simulink model "Tariq"  (Simulink 10.0)
settings: Solver=ode45  StartTime=0.0  StopTime=10  RelTol=1e-3  EnableMultiTasking=on
undefined symbols (not defined in the file): B, f, J, Lm, Lr, Ls, P, Rr, Rs, Vm, We
libraries: simulink x2
settings Model: Creator=Administrator  LastModifiedBy=unknown
settings DataIOCC: LimitDataPoints=on  SignalLoggingSaveFormat=ModelDataLogs
settings OptimizationCC: ExpressionDepthLimit=2147483647  InitFltsAndDblsToZero=on
settings DebuggingCC: SaveWithParameterizedLinksMsg=none  SignalResolutionControl=TryResolveAllWithWarning  SolverPrmCheckMsg=warning  FcnCallInpInsideContextMsg=warning  StateNameClashWarn=warning
settings GRTTargetCC: TargetFcnLib=ansi_tfl_tmw.mat
settings ConfigComp: CovExternalEMLEnable=off

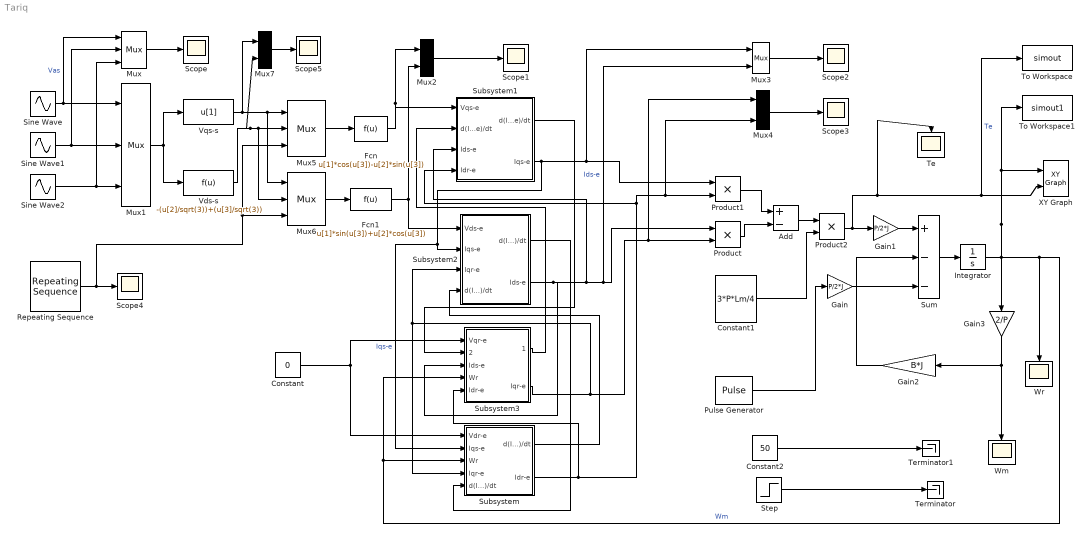
== system Tariq ==
  Add : Sum  Inputs=+-
  Constant : Constant  Value=0
  Constant1 : Constant  Value=3*P*Lm/4
  Constant2 : Constant  Value=50
  Fcn : Fcn  Expr=u[1]*cos(u[3])-u[2]*sin(u[3])
  Fcn1 : Fcn  Expr=u[1]*sin(u[3])+u[2]*cos(u[3])
  Gain : Gain  Gain=P/2*J
  Gain1 : Gain  Gain=P/2*J
  Gain2 : Gain  Gain=B*J
  Gain3 : Gain  Gain=2/P
  Integrator : Integrator
  Mux{,1,5..6} (4 alike) : Mux  Inputs=3
      settings: DisplayOption=signals
  Mux{2..4,7} (4 alike) : Mux  Inputs=2
      settings: DisplayOption=signals
  Product : Product  RndMeth=Zero
  Product1 : Product  RndMeth=Zero
  Product2 : Product  RndMeth=Zero
  Pulse Generator : DiscretePulseGenerator  Amplitude=40  Period=10  PulseWidth=5  PhaseDelay=4
  Repeating Sequence : simulink/Sources/Repeating Sequence  SystemSampleTime=-1  rep_seq_t=[0 1/f]  rep_seq_y=[0 2*pi]
  Scope{,1..5} (6 alike) : Scope
  Sine Wave : Sin  Amplitude=Vm  Frequency=2*pi*50  Phase=pi/2  SampleTime=0
  Sine Wave1 : Sin  Amplitude=Vm  Frequency=2*pi*50  Phase=(pi/2)-(2*pi/3)  SampleTime=0
  Sine Wave2 : Sin  Amplitude=Vm  Frequency=2*pi*50  Phase=(pi/2)+(2*pi/3)  SampleTime=0
  Step : Step  Time=0.5  After=40  SampleTime=0
  Subsystem : Subsystem
  Subsystem1 : Subsystem
  Subsystem2 : Subsystem
  Subsystem3 : Subsystem
  Sum : Sum  Inputs=+--
  Te : Scope
  Terminator : Terminator
  Terminator1 : Terminator
  To Workspace : ToWorkspace  VariableName=simout  SaveFormat=Structure  SampleTime=-1
  To Workspace1 : ToWorkspace  VariableName=simout1  SaveFormat=Structure  SampleTime=-1
  Vds-s : Fcn  Expr=-(u[2]/sqrt(3))+(u[3]/sqrt(3))
  Vqs-s : Fcn  Expr=u[1]
  Wm : Scope
  Wr : Scope
  XY Graph : simulink/Sinks/XY Graph  SystemSampleTime=-1  xmin=0  xmax=350  ymin=-400  ymax=400  st=-1
  wires:
  Mux/1 -> Scope/1
  Mux2/1 -> Scope1/1
  Mux3/1 -> Scope2/1
  Mux4/1 -> Scope3/1
  Product1/1 -> Add/1
  Product/1 -> Add/2
  Add/1 -> Product2/1
  Constant1/1 -> Product2/2
  Product2/1 -> Gain1/1, XY Graph/2, To Workspace/1, Te/1  "Te"
  Gain1/1 -> Sum/1
  Gain/1 -> Sum/3
  Pulse Generator/1 -> Gain/1
  Sum/1 -> Integrator/1
  Integrator/1 -> XY Graph/1, To Workspace1/1, Gain3/1, Subsystem3/4(Wr), Subsystem/3(Wr), Wr/1  "Wm"
  Gain2/1 -> Sum/2
  Gain3/1 -> Wm/1, Gain2/1
  Constant2/1 -> Terminator1/1
  Step/1 -> Terminator/1
  Repeating Sequence/1 -> Scope4/1, Mux5/3, Mux6/3
  Sine Wave/1 -> Mux1/1, Mux/1  "Vas"
  Sine Wave1/1 -> Mux1/2, Mux/2
  Sine Wave2/1 -> Mux1/3, Mux/3
  Mux1/1 -> Vqs-s/1, Vds-s/1
  Vqs-s/1 -> Mux5/1, Mux6/1, Mux7/1
  Vds-s/1 -> Mux5/2, Mux6/2, Mux7/2
  Mux5/1 -> Fcn/1
  Mux6/1 -> Fcn1/1
  Fcn/1 -> Mux2/1, Subsystem1/1(Vqs-e)
  Fcn1/1 -> Mux2/2, Subsystem2/1(Vds-e)
  Mux7/1 -> Scope5/1
  Subsystem1/2(Iqs-e) -> Subsystem2/2(Iqs-e), Subsystem/2(Iqs-e), Product1/1, Mux3/1  "Iqs-e"
  Subsystem/2(Idr-e) -> Subsystem1/4(Idr-e), Product1/2, Mux4/2, Subsystem3/5(Idr-e)
  Subsystem2/2(Ids-e) -> Subsystem1/3(Ids-e), Product/1, Mux3/2, Subsystem3/3(Ids-e)  "Ids-e"
  Subsystem3/2(Iqr-e) -> Subsystem2/3(Iqr-e), Subsystem/4(Iqr-e), Product/2, Mux4/1
  Subsystem/1(d(Idr-e)/dt) -> Subsystem2/4(d(Idr-e)/dt)
  Constant/1 -> Subsystem3/1(Vqr-e), Subsystem/1(Vdr-e)
  Subsystem1/1(d(Iqs-e)/dt) -> Subsystem3/2(d(Iqs-e)/dt)
  Subsystem2/1(d(Ids-e)/dt) -> Subsystem/5(d(Ids-e)/dt)
  Subsystem3/1(d(Iqr-e)/dt) -> Subsystem1/2(d(Iqr-e)/dt)

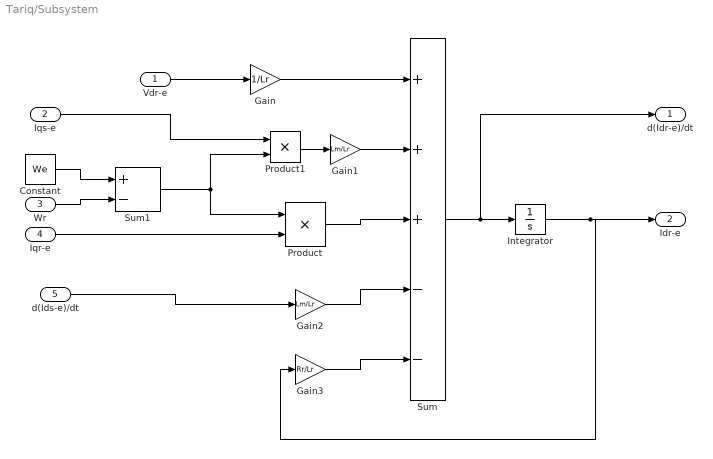
== system Tariq/Subsystem ==
  Vdr-e : Inport
  Iqs-e : Inport  Port=2
  Wr : Inport  Port=3
  Iqr-e : Inport  Port=4
  d(Ids-e)/dt : Inport  Port=5
  Constant : Constant  Value=We
  Gain : Gain  Gain=1/Lr
  Gain1 : Gain  Gain=Lm/Lr
  Gain2 : Gain  Gain=Lm/Lr
  Gain3 : Gain  Gain=Rr/Lr
  Integrator : Integrator
  Product : Product  RndMeth=Zero
  Product1 : Product  RndMeth=Zero
  Sum : Sum  Inputs=+++--
  Sum1 : Sum  Inputs=+-
  d(Idr-e)/dt : Outport
  Idr-e : Outport  Port=2
  wires:
  Gain/1 -> Sum/1
  Vdr-e/1 -> Gain/1
  Gain1/1 -> Sum/2
  Product1/1 -> Gain1/1
  Sum1/1 -> Product1/2, Product/1
  Constant/1 -> Sum1/1
  Wr/1 -> Sum1/2
  Iqs-e/1 -> Product1/1
  Iqr-e/1 -> Product/2
  Product/1 -> Sum/3
  Gain2/1 -> Sum/4
  d(Ids-e)/dt/1 -> Gain2/1
  Sum/1 -> Integrator/1, d(Idr-e)/dt/1
  Integrator/1 -> Idr-e/1, Gain3/1
  Gain3/1 -> Sum/5

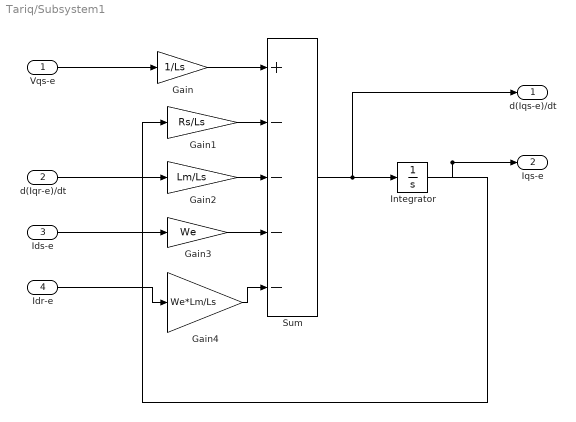
== system Tariq/Subsystem1 ==
  Vqs-e : Inport
  d(Iqr-e)/dt : Inport  Port=2
  Ids-e : Inport  Port=3
  Idr-e : Inport  Port=4
  Gain : Gain  Gain=1/Ls
  Gain1 : Gain  Gain=Rs/Ls
  Gain2 : Gain  Gain=Lm/Ls
  Gain3 : Gain  Gain=We
  Gain4 : Gain  Gain=We*Lm/Ls
  Integrator : Integrator
  Sum : Sum  Inputs=+----
  d(Iqs-e)/dt : Outport
  Iqs-e : Outport  Port=2
  wires:
  Vqs-e/1 -> Gain/1
  Gain/1 -> Sum/1
  Gain1/1 -> Sum/2
  Gain2/1 -> Sum/3
  Sum/1 -> Integrator/1, d(Iqs-e)/dt/1
  d(Iqr-e)/dt/1 -> Gain2/1
  Integrator/1 -> Iqs-e/1, Gain1/1
  Gain3/1 -> Sum/4
  Ids-e/1 -> Gain3/1
  Gain4/1 -> Sum/5
  Idr-e/1 -> Gain4/1

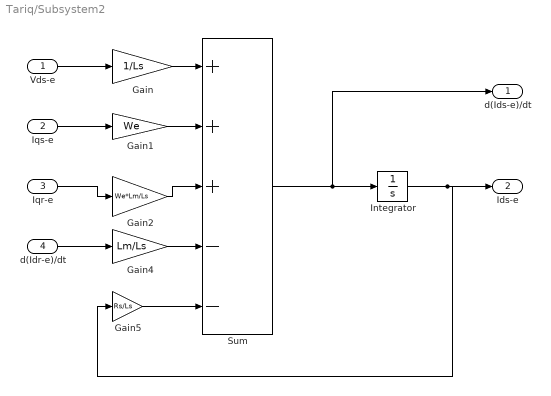
== system Tariq/Subsystem2 ==
  Vds-e : Inport
  Iqs-e : Inport  Port=2
  Iqr-e : Inport  Port=3
  d(Idr-e)/dt : Inport  Port=4
  Gain : Gain  Gain=1/Ls
  Gain1 : Gain  Gain=We
  Gain2 : Gain  Gain=We*Lm/Ls
  Gain4 : Gain  Gain=Lm/Ls
  Gain5 : Gain  Gain=Rs/Ls
  Integrator : Integrator
  Sum : Sum  Inputs=+++--
  d(Ids-e)/dt : Outport
  Ids-e : Outport  Port=2
  wires:
  Gain/1 -> Sum/1
  Vds-e/1 -> Gain/1
  Gain1/1 -> Sum/2
  Iqs-e/1 -> Gain1/1
  Iqr-e/1 -> Gain2/1
  Gain2/1 -> Sum/3
  d(Idr-e)/dt/1 -> Gain4/1
  Gain4/1 -> Sum/4
  Gain5/1 -> Sum/5
  Sum/1 -> Integrator/1, d(Ids-e)/dt/1
  Integrator/1 -> Ids-e/1, Gain5/1

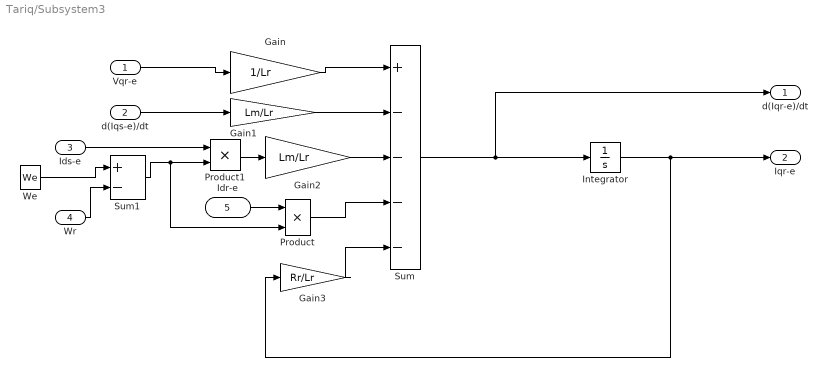
== system Tariq/Subsystem3 ==
  Vqr-e : Inport
  d(Iqs-e)/dt : Inport  Port=2
  Ids-e : Inport  Port=3
  Wr : Inport  Port=4
  Idr-e : Inport  Port=5
  Gain : Gain  Gain=1/Lr
  Gain1 : Gain  Gain=Lm/Lr
  Gain2 : Gain  Gain=Lm/Lr
  Gain3 : Gain  Gain=Rr/Lr
  Integrator : Integrator
  Product : Product  RndMeth=Zero
  Product1 : Product  RndMeth=Zero
  Sum : Sum  Inputs=+----
  Sum1 : Sum  Inputs=+-
  We : Constant  Value=We
  d(Iqr-e)/dt : Outport
  Iqr-e : Outport  Port=2
  wires:
  Gain/1 -> Sum/1
  Gain1/1 -> Sum/2
  Sum/1 -> Integrator/1, d(Iqr-e)/dt/1
  Integrator/1 -> Iqr-e/1, Gain3/1
  Vqr-e/1 -> Gain/1
  d(Iqs-e)/dt/1 -> Gain1/1
  Ids-e/1 -> Product1/1
  Product1/1 -> Gain2/1
  Gain2/1 -> Sum/3
  Sum1/1 -> Product1/2, Product/2
  Wr/1 -> Sum1/2
  Product/1 -> Sum/4
  Idr-e/1 -> Product/1
  Gain3/1 -> Sum/5
  We/1 -> Sum1/1
